simulink model "untitled1"  (R2018a)
settings: Solver=VariableStepAuto  StartTime=0.0  StopTime=10.0  RelTol=1e-3
settings Model: Creator=9920103168  LastModifiedBy=9920103168

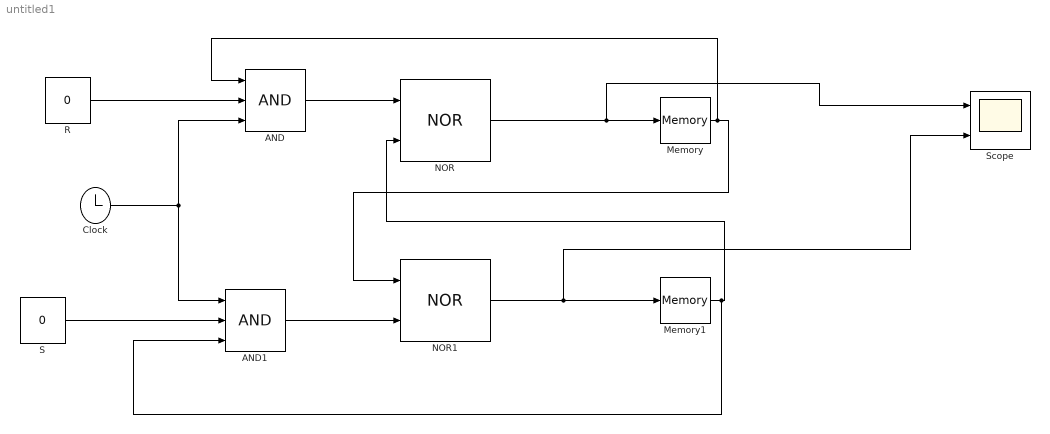
== system untitled1 ==
  AND : Logic  Inputs=3  IconShape=distinctive  AllPortsSameDT=off  OutDataTypeStr=boolean
  AND1 : Logic  Inputs=3  IconShape=distinctive  AllPortsSameDT=off  OutDataTypeStr=boolean
  Clock : Clock
  Memory : Memory
  Memory1 : Memory
  NOR : Logic  Operator=NOR  IconShape=distinctive  AllPortsSameDT=off  OutDataTypeStr=boolean
  NOR1 : Logic  Operator=NOR  IconShape=distinctive  AllPortsSameDT=off  OutDataTypeStr=boolean
  R : Constant  Value=0
  S : Constant  Value=0
  Scope : Scope  NumInputPorts=2
  wires:
  NOR1/1 -> Scope/2, Memory1/1
  Memory/1 -> AND/1, NOR1/1
  Memory1/1 -> AND1/3, NOR/2
  AND/1 -> NOR/1
  AND1/1 -> NOR1/2
  R/1 -> AND/2
  S/1 -> AND1/2
  Clock/1 -> AND1/1, AND/3
  NOR/1 -> Scope/1, Memory/1
